simulink model "gm_DUALportRAMinterface_v3"  (R2024a)
settings: Solver=FixedStepDiscrete  StartTime=0.0  StopTime=20  RelTol=1e-3
undefined symbols (not defined in the file or in its folder): magnitude, Ts
libraries: hdlsllib x226, hdlmdlgenlib x102, embmathops x6, simulink x1, dsphdlxfrm2 x1
(part 1 of 6)
settings Model: Creator=Simon  LastModifiedBy=Simon
settings OptimizationCC: BlockReduction=off  ConditionallyExecuteInputs=off  DefaultParameterBehavior=Inlined  InheritOutputTypeSmallerThanSingle=on
settings DebuggingCC: AlgebraicLoopMsg=error  InheritedTsInSrcMsg=none  SingleTaskRateTransMsg=error  UnconnectedInputMsg=warning  UnconnectedOutputMsg=warning  UnconnectedLineMsg=warning
settings HardwareCC: ProdBitPerPointer=32  ProdBitPerSizeT=32  ProdBitPerPtrDiffT=32  ProdLargestAtomicFloat=None  ProdIntDivRoundTo=Undefined  ProdEndianess=Unspecified  ProdWordSize=32  ProdHWDeviceType=ASIC/FPGA->ASIC/FPGA  TargetBitPerPointer=64  TargetBitPerSizeT=64  TargetBitPerPtrDiffT=64  TargetLongLongMode=on  TargetIntDivRoundTo=Zero  TargetEndianess=LittleEndian  TargetWordSize=64  TargetHWDeviceType=Custom Processor->MATLAB Host Computer  ProdEqTarget=off

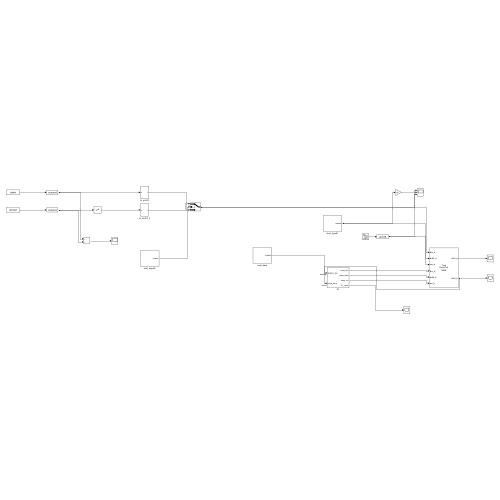
[thumbnail: Simulink's stored preview of the top-level diagram]
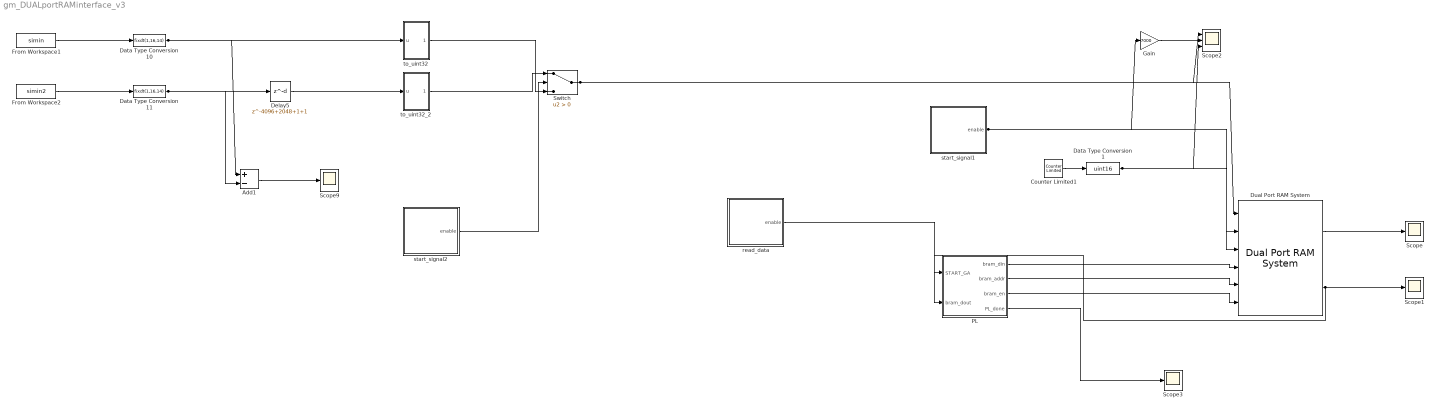
== system gm_DUALportRAMinterface_v3 ==
  Add1 : Sum  Inputs=+-
  Counter Limited1 : simulink/Sources/Counter Limited  uplimit=14000  tsamp=Ts
  Data Type Conversion1 : DataTypeConversion  OutDataTypeStr=uint16  SaturateOnIntegerOverflow=off  RndMeth=Floor
  Data Type Conversion10 : DataTypeConversion  OutDataTypeStr=fixdt(1,16,14)  SaturateOnIntegerOverflow=off  RndMeth=Floor
  Data Type Conversion11 : DataTypeConversion  OutDataTypeStr=fixdt(1,16,14)  SaturateOnIntegerOverflow=off  RndMeth=Floor
  Delay5 : Delay  DelayLength=4096+2048+1+1  InitialCondition=0  SampleTime=Ts
  Dual Port RAM System : hdlsllib/HDL RAMs/Dual Port RAM System  RAMType=True dual port  AsyncRead=off  WriteOutputValue=New data  RAMInitialValue=0  allowBusInputs=off  WritesHaveOutput=on  NumReads=0  NumWrites=1  SimulateUsing=Code generation
  From Workspace1 : FromWorkspace  VariableName=simin  SampleTime=Ts
  From Workspace2 : FromWorkspace  VariableName=simin2  SampleTime=Ts
  Gain : Gain  Gain=7000
  PL : Subsystem
  Scope{,1,3,9} (4 alike) : Scope
  Scope2 : Scope  NumInputPorts=3
  Switch : Switch  Criteria=u2 > Threshold  SaturateOnIntegerOverflow=off  InputSameDT=off  OutDataTypeStr=Inherit: Same as first input
  read_data : Subsystem
  start_signal1 : Subsystem
  start_signal2 : Subsystem
  to_uint32 : Subsystem
  to_uint32_2 : Subsystem
  wires:
  PL/4(PL_done) -> Scope3/1
  Data Type Conversion10/1 -> to_uint32/1(u), Add1/1
  Add1/1 -> Scope9/1
  Data Type Conversion11/1 -> Add1/2, Delay5/1
  Switch/1 -> Dual Port RAM System/1, Scope2/1
  Delay5/1 -> to_uint32_2/1(u)
  start_signal2/1(enable) -> Switch/2
  to_uint32_2/1(Out1) -> Switch/1
  to_uint32/1(Out1) -> Switch/3
  From Workspace2/1 -> Data Type Conversion11/1
  From Workspace1/1 -> Data Type Conversion10/1
  Dual Port RAM System/2 -> PL/2(bram_dout), Scope1/1
  read_data/1(enable) -> PL/1(START_GA)
  Gain/1 -> Scope2/2
  PL/3(bram_en) -> Dual Port RAM System/6
  PL/2(bram_addr) -> Dual Port RAM System/5
  PL/1(bram_din) -> Dual Port RAM System/4
  start_signal1/1(enable) -> Gain/1, Dual Port RAM System/3
  Data Type Conversion1/1 -> Dual Port RAM System/2, Scope2/3
  Counter Limited1/1 -> Data Type Conversion1/1
  Dual Port RAM System/1 -> Scope/1

== system gm_DUALportRAMinterface_v3/PL ==
  START_GA : Inport  OutDataTypeStr=boolean  PortDimensions=1  SampleTime=3.00000003e-08
  bram_dout : Inport  Port=2  OutDataTypeStr=uint32  PortDimensions=1  SampleTime=3.00000003e-08
  Bit Shift18 : hdlsllib/Logic and Bit Operations/Bit Shift  mode=Shift Right Logical  N=double(14)
  Chart : Subsystem
  Data Type Conversion2 : DataTypeConversion  OutDataTypeStr=uint32  SampleTime=3.00000003e-08  SaturateOnIntegerOverflow=off  RndMeth=Floor
  Data Type Conversion8 : DataTypeConversion  OutDataTypeStr=fixdt(0, 30, 14)  SampleTime=3.00000003e-08  SaturateOnIntegerOverflow=off  RndMeth=Floor
  Data Type Conversion9 : DataTypeConversion  OutDataTypeStr=fixdt(1, 16, 14)  SampleTime=3.00000003e-08  SaturateOnIntegerOverflow=off  RndMeth=Floor
  Delay : Delay  DelayLength=double(16)  InitialCondition=0  SampleTime=3.00000003e-08
  From{1..4,6,10..11} (7 alike) : hdlmdlgenlib/Buffer
  Goto{,1..5} (6 alike) : hdlmdlgenlib/Buffer
  Multiport Switch : MultiPortSwitch  DataPortOrder=Specify indices  Inputs=8  DataPortIndices={ double(0) double(1) double(2) double(3) double(4) double(5) double(6) double(7)}  DataPortForDefault=Additional data port  DiagnosticForDefault=None  OutDataTypeStr=uint32  SampleTime=3.00000003e-08  SaturateOnIntegerOverflow=off  InputSameDT=off
  index_counter : Subsystem
  integration_block1 : Subsystem
  t : Demux  Outputs=7
  to_uint32_1 : Subsystem
  to_uint32_2 : Subsystem
  to_uint32_3 : Subsystem
  to_uint32_4 : Subsystem
  to_uint32_5 : Subsystem
  to_uint32_6 : Subsystem
  bram_din : Outport  SampleTime=3.00000003e-08
  bram_addr : Outport  Port=2  SampleTime=3.00000003e-08
  bram_en : Outport  Port=3  SampleTime=3.00000003e-08
  PL_done : Outport  Port=4  SampleTime=3.00000003e-08
  wires:
  START_GA/1 -> integration_block1/3(start_ga), Chart/2(GPIO)
  bram_dout/1 -> Data Type Conversion8/1
  Bit Shift18/1 -> Data Type Conversion9/1
  Chart/3(write_enable) -> Goto4/1
  Data Type Conversion2/1 -> Multiport Switch/10, Multiport Switch/9, Multiport Switch/2
  Data Type Conversion8/1 -> Bit Shift18/1
  Data Type Conversion9/1 -> integration_block1/1(data_in), integration_block1/2(data_in1)
  Delay/1 -> Goto3/1
  From1/1 -> bram_addr/1
  From2/1 -> bram_en/1
  From3/1 -> PL_done/1
  From4/1 -> bram_din/1
  From6/1 -> Multiport Switch/1
  Multiport Switch/1 -> Goto/1
  index_counter/1(index_counter) -> Goto5/1, Chart/3(counter)
  integration_block1/1(ga_done) -> Delay/1, Chart/1(GA_done)
  integration_block1/2(elite_individual) -> t/1
  to_uint32_1/1(Out1) -> Multiport Switch/3
  to_uint32_2/1(Out1) -> Multiport Switch/4
  to_uint32_3/1(Out1) -> Multiport Switch/5
  to_uint32_4/1(Out1) -> Multiport Switch/6
  to_uint32_5/1(Out1) -> Multiport Switch/7
  to_uint32_6/1(Out1) -> Multiport Switch/8
  Goto5/1 -> From6/1, From1/1
  Goto4/1 -> From2/1
  Goto3/1 -> From3/1
  Goto/1 -> From4/1
  t/1 -> Data Type Conversion2/1
  t/2 -> to_uint32_1/1(u_port)
  t/3 -> to_uint32_2/1(u_port)
  t/4 -> to_uint32_3/1(u_port)
  t/5 -> to_uint32_4/1(u_port)
  t/6 -> to_uint32_5/1(u_port)
  t/7 -> to_uint32_6/1(u_port)
  From10/1 -> index_counter/2(In2)
  From11/1 -> index_counter/1(In1)
  Goto2/1 -> From10/1
  Goto1/1 -> From11/1
  Chart/1(counter_increment) -> Goto1/1
  Chart/2(counter_reset) -> Goto2/1

== system gm_DUALportRAMinterface_v3/read_data ==
  Data Type Conversion29 : DataTypeConversion  OutDataTypeStr=boolean  SaturateOnIntegerOverflow=off  RndMeth=Floor
  Delay2 : Delay  DelayLength=1  InitialCondition=0  SampleTime=Ts
  Gain : Gain
  Step1 : Step  Time=Ts*14000  SampleTime=Ts
  XOR1 : Logic  Operator=XOR  IconShape=distinctive  AllPortsSameDT=off  OutDataTypeStr=boolean
  enable : Outport
  wires:
  Data Type Conversion29/1 -> enable/1
  Gain/1 -> Data Type Conversion29/1
  Delay2/1 -> XOR1/2
  Step1/1 -> XOR1/1, Delay2/1
  XOR1/1 -> Gain/1

== system gm_DUALportRAMinterface_v3/start_signal1 ==
  Data Type Conversion29 : DataTypeConversion  OutDataTypeStr=boolean  SaturateOnIntegerOverflow=off  RndMeth=Floor
  Delay2 : Delay  DelayLength=(4096+2048+1+1)*2  InitialCondition=0  SampleTime=Ts
  Gain : Gain
  Step1 : Step  Time=Ts*0  SampleTime=Ts
  XOR1 : Logic  Operator=XOR  IconShape=distinctive  AllPortsSameDT=off  OutDataTypeStr=boolean
  enable : Outport
  wires:
  XOR1/1 -> Gain/1
  Step1/1 -> Delay2/1, XOR1/1
  Delay2/1 -> XOR1/2
  Gain/1 -> Data Type Conversion29/1
  Data Type Conversion29/1 -> enable/1

== system gm_DUALportRAMinterface_v3/start_signal2 ==
  Data Type Conversion29 : DataTypeConversion  OutDataTypeStr=boolean  SaturateOnIntegerOverflow=off  RndMeth=Floor
  Delay2 : Delay  DelayLength=(4096+2048+1+1)*2  InitialCondition=0  SampleTime=Ts
  Gain : Gain
  Step1 : Step  Time=Ts*(4096+2048+1+1)  SampleTime=Ts
  XOR1 : Logic  Operator=XOR  IconShape=distinctive  AllPortsSameDT=off  OutDataTypeStr=boolean
  enable : Outport
  wires:
  Data Type Conversion29/1 -> enable/1
  Gain/1 -> Data Type Conversion29/1
  Delay2/1 -> XOR1/2
  Step1/1 -> XOR1/1, Delay2/1
  XOR1/1 -> Gain/1

== system gm_DUALportRAMinterface_v3/to_uint32 ==
  u : Inport
  Bit Concat2 : hdlsllib/Logic and Bit Operations/Bit Concat  numInputs=16
  Bit Shift19 : hdlsllib/Logic and Bit Operations/Bit Shift  mode=Shift Left Logical  N=1
  Bit Shift20 : hdlsllib/Logic and Bit Operations/Bit Shift  mode=Shift Left Logical  N=10
  Bit Shift21 : hdlsllib/Logic and Bit Operations/Bit Shift  mode=Shift Right Logical  N=1
  Bit Shift22 : hdlsllib/Logic and Bit Operations/Bit Shift  mode=Shift Left Logical  N=11
  Bit Shift23 : hdlsllib/Logic and Bit Operations/Bit Shift  mode=Shift Left Logical  N=12
  Bit Shift24 : hdlsllib/Logic and Bit Operations/Bit Shift  mode=Shift Left Logical  N=13
  Bit Shift25 : hdlsllib/Logic and Bit Operations/Bit Shift  mode=Shift Left Logical  N=14
  Bit Shift26 : hdlsllib/Logic and Bit Operations/Bit Shift  mode=Shift Left Logical  N=2
  Bit Shift27 : hdlsllib/Logic and Bit Operations/Bit Shift  mode=Shift Left Logical  N=3
  Bit Shift28 : hdlsllib/Logic and Bit Operations/Bit Shift  mode=Shift Left Logical  N=4
  Bit Shift29 : hdlsllib/Logic and Bit Operations/Bit Shift  mode=Shift Left Logical  N=5
  Bit Shift30 : hdlsllib/Logic and Bit Operations/Bit Shift  mode=Shift Left Logical  N=6
  Bit Shift31 : hdlsllib/Logic and Bit Operations/Bit Shift  mode=Shift Left Logical  N=7
  Bit Shift32 : hdlsllib/Logic and Bit Operations/Bit Shift  mode=Shift Left Logical  N=8
  Bit Shift33 : hdlsllib/Logic and Bit Operations/Bit Shift  mode=Shift Left Logical  N=9
  Data Type Conversion{12..16,26,34..43} (16 alike) : DataTypeConversion  OutDataTypeStr=fixdt(0,1,0)  SaturateOnIntegerOverflow=off  RndMeth=Floor
  Data Type Conversion44 : DataTypeConversion  OutDataTypeStr=uint32  SaturateOnIntegerOverflow=off  RndMeth=Floor
  Out1 : Outport
  wires:
  Data Type Conversion14/1 -> Bit Concat2/10
  Bit Concat2/1 -> Data Type Conversion44/1
  Bit Shift26/1 -> Data Type Conversion35/1
  Bit Shift21/1 -> Data Type Conversion13/1
  Bit Shift28/1 -> Data Type Conversion26/1
  Data Type Conversion37/1 -> Bit Concat2/16
  Bit Shift29/1 -> Data Type Conversion16/1
  Bit Shift23/1 -> Data Type Conversion39/1
  Data Type Conversion41/1 -> Bit Concat2/12
  Bit Shift24/1 -> Data Type Conversion38/1
  Bit Shift33/1 -> Data Type Conversion42/1
  Data Type Conversion16/1 -> Bit Concat2/7
  Data Type Conversion43/1 -> Bit Concat2/9
  Data Type Conversion34/1 -> Bit Concat2/5
  Data Type Conversion39/1 -> Bit Concat2/14
  Bit Shift32/1 -> Data Type Conversion14/1
  Data Type Conversion12/1 -> Bit Concat2/2
  Bit Shift30/1 -> Data Type Conversion15/1
  Data Type Conversion15/1 -> Bit Concat2/8
  Bit Shift25/1 -> Data Type Conversion37/1
  Data Type Conversion38/1 -> Bit Concat2/15
  Bit Shift19/1 -> Data Type Conversion36/1
  Data Type Conversion42/1 -> Bit Concat2/11
  Data Type Conversion35/1 -> Bit Concat2/4
  Data Type Conversion44/1 -> Out1/1
  Data Type Conversion26/1 -> Bit Concat2/6
  Bit Shift31/1 -> Data Type Conversion43/1
  Data Type Conversion40/1 -> Bit Concat2/13
  Data Type Conversion13/1 -> Bit Concat2/1
  Bit Shift20/1 -> Data Type Conversion41/1
  u/1 -> Bit Shift25/1, Bit Shift24/1, Bit Shift23/1, Bit Shift22/1, Bit Shift20/1, Bit Shift33/1, Bit Shift32/1, Bit Shift31/1, Bit Shift30/1, Bit Shift29/1, Bit Shift28/1, Bit Shift27/1, Bit Shift26/1, Bit Shift19/1, Data Type Conversion12/1, Bit Shift21/1
  Data Type Conversion36/1 -> Bit Concat2/3
  Bit Shift27/1 -> Data Type Conversion34/1
  Bit Shift22/1 -> Data Type Conversion40/1

== system gm_DUALportRAMinterface_v3/to_uint32_2 ==
  u : Inport
  Bit Concat2 : hdlsllib/Logic and Bit Operations/Bit Concat  numInputs=16
  Bit Shift19 : hdlsllib/Logic and Bit Operations/Bit Shift  mode=Shift Left Logical  N=1
  Bit Shift20 : hdlsllib/Logic and Bit Operations/Bit Shift  mode=Shift Left Logical  N=10
  Bit Shift21 : hdlsllib/Logic and Bit Operations/Bit Shift  mode=Shift Right Logical  N=1
  Bit Shift22 : hdlsllib/Logic and Bit Operations/Bit Shift  mode=Shift Left Logical  N=11
  Bit Shift23 : hdlsllib/Logic and Bit Operations/Bit Shift  mode=Shift Left Logical  N=12
  Bit Shift24 : hdlsllib/Logic and Bit Operations/Bit Shift  mode=Shift Left Logical  N=13
  Bit Shift25 : hdlsllib/Logic and Bit Operations/Bit Shift  mode=Shift Left Logical  N=14
  Bit Shift26 : hdlsllib/Logic and Bit Operations/Bit Shift  mode=Shift Left Logical  N=2
  Bit Shift27 : hdlsllib/Logic and Bit Operations/Bit Shift  mode=Shift Left Logical  N=3
  Bit Shift28 : hdlsllib/Logic and Bit Operations/Bit Shift  mode=Shift Left Logical  N=4
  Bit Shift29 : hdlsllib/Logic and Bit Operations/Bit Shift  mode=Shift Left Logical  N=5
  Bit Shift30 : hdlsllib/Logic and Bit Operations/Bit Shift  mode=Shift Left Logical  N=6
  Bit Shift31 : hdlsllib/Logic and Bit Operations/Bit Shift  mode=Shift Left Logical  N=7
  Bit Shift32 : hdlsllib/Logic and Bit Operations/Bit Shift  mode=Shift Left Logical  N=8
  Bit Shift33 : hdlsllib/Logic and Bit Operations/Bit Shift  mode=Shift Left Logical  N=9
  Data Type Conversion{12..16,26,34..43} (16 alike) : DataTypeConversion  OutDataTypeStr=fixdt(0,1,0)  SaturateOnIntegerOverflow=off  RndMeth=Floor
  Data Type Conversion44 : DataTypeConversion  OutDataTypeStr=uint32  SaturateOnIntegerOverflow=off  RndMeth=Floor
  Out1 : Outport
  wires:
  Bit Shift22/1 -> Data Type Conversion40/1
  Bit Shift27/1 -> Data Type Conversion34/1
  Data Type Conversion36/1 -> Bit Concat2/3
  u/1 -> Bit Shift21/1, Data Type Conversion12/1, Bit Shift19/1, Bit Shift26/1, Bit Shift27/1, Bit Shift28/1, Bit Shift29/1, Bit Shift30/1, Bit Shift31/1, Bit Shift32/1, Bit Shift33/1, Bit Shift20/1, Bit Shift22/1, Bit Shift23/1, Bit Shift24/1, Bit Shift25/1
  Bit Shift20/1 -> Data Type Conversion41/1
  Data Type Conversion13/1 -> Bit Concat2/1
  Data Type Conversion40/1 -> Bit Concat2/13
  Bit Shift31/1 -> Data Type Conversion43/1
  Data Type Conversion26/1 -> Bit Concat2/6
  Data Type Conversion44/1 -> Out1/1
  Data Type Conversion35/1 -> Bit Concat2/4
  Data Type Conversion42/1 -> Bit Concat2/11
  Bit Shift19/1 -> Data Type Conversion36/1
  Data Type Conversion38/1 -> Bit Concat2/15
  Bit Shift25/1 -> Data Type Conversion37/1
  Data Type Conversion15/1 -> Bit Concat2/8
  Bit Shift30/1 -> Data Type Conversion15/1
  Data Type Conversion12/1 -> Bit Concat2/2
  Bit Shift32/1 -> Data Type Conversion14/1
  Data Type Conversion39/1 -> Bit Concat2/14
  Data Type Conversion34/1 -> Bit Concat2/5
  Data Type Conversion43/1 -> Bit Concat2/9
  Data Type Conversion16/1 -> Bit Concat2/7
  Bit Shift33/1 -> Data Type Conversion42/1
  Bit Shift24/1 -> Data Type Conversion38/1
  Data Type Conversion41/1 -> Bit Concat2/12
  Bit Shift23/1 -> Data Type Conversion39/1
  Bit Shift29/1 -> Data Type Conversion16/1
  Data Type Conversion37/1 -> Bit Concat2/16
  Bit Shift28/1 -> Data Type Conversion26/1
  Bit Shift21/1 -> Data Type Conversion13/1
  Bit Shift26/1 -> Data Type Conversion35/1
  Bit Concat2/1 -> Data Type Conversion44/1
  Data Type Conversion14/1 -> Bit Concat2/10

== system gm_DUALportRAMinterface_v3/PL/Chart ==
  GA_done : Inport  OutDataTypeStr=boolean  PortDimensions=1  SampleTime=3.00000003e-08
  GPIO : Inport  Port=2  OutDataTypeStr=boolean  PortDimensions=1  SampleTime=3.00000003e-08
  counter : Inport  Port=3  OutDataTypeStr=uint16  PortDimensions=1  SampleTime=3.00000003e-08
  Chart : Stateflow chart  TreatAsAtomicUnit=on
      settings: PortSchema="{\"entries\":[{\"content\":{\"sides\":[{\"content\":{\"connectorIds\":[\"In2\",\"In3\"]},\"type\":\"ConnectorPlacement.EquallySpacedRectSide\",\"uuid\":\"f3ce331f-c708-4668-a9cb-fb327ea74ab5\"},{\"content\":{\"connectorIds\":[\"Out1\",\"Out2\",\"Out3\"],\"side\":\"RIGHT\"},\"type\":\"ConnectorPlacement.EquallySpacedRectSide\",\"uuid\":\"3766927a-abff-497d-9544-2098881ba174\"},{\"content\":{\"side\":\"TOP\"},\"type\":\"ConnectorPlacement.EquallySpacedRectSide\",\"uuid\":\"ebfe3d64-ee7d-4953-a6ba-e7e40988decf\"},{\"content\":{\"connectorIds\":[\"In1\"],\"side\":\"BOTTOM\"},\"type\":\"ConnectorPlacement.EquallySpacedRectSide\",\"uuid\":\"f39ceaf8-4df7-4e40-9de5-da7597831fb4\"}]},\"type\":\"ConnectorPlacement.EquallySpacedConnector\",\"uuid\":\"89f60450-5933-42bb-b72b-5f8ec55483e0\"}],\"packageUris\":[\"http://schema.mathworks.com/mf0/Connector/R2020b\"],\"version\":\"1.0\"}"
  counter_increment : Outport  SampleTime=3.00000003e-08
  counter_reset : Outport  Port=2  SampleTime=3.00000003e-08
  write_enable : Outport  Port=3  SampleTime=3.00000003e-08
  wires:
  GA_done/1 -> Chart/1(GA_done)
  GPIO/1 -> Chart/2(GPIO)
  counter/1 -> Chart/3(counter)
  Chart/1(counter_increment) -> counter_increment/1
  Chart/2(counter_reset) -> counter_reset/1
  Chart/3(write_enable) -> write_enable/1

== system gm_DUALportRAMinterface_v3/PL/index_counter ==
  In1 : Inport  OutDataTypeStr=boolean  PortDimensions=1  SampleTime=3.00000003e-08
  In2 : Inport  Port=2  OutDataTypeStr=boolean  PortDimensions=1  SampleTime=3.00000003e-08
  Add : Sum  OutDataTypeStr=uint16
  Constant18 : Constant  OutDataTypeStr=fixdt(0,16,0)  SampleTime=Ts
  Constant19 : Constant  Value=0  OutDataTypeStr=fixdt(0,16,0)  SampleTime=Ts
  Constant20 : Constant  Value=0  OutDataTypeStr=uint16  SampleTime=Ts
  Delay : Delay  DelayLength=1  InitialCondition=0  SampleTime=Ts
  Switch : Switch  Criteria=u2 > Threshold  OutDataTypeStr=uint16  SaturateOnIntegerOverflow=off  InputSameDT=off
  Switch8 : Switch  Criteria=u2 > Threshold  OutDataTypeStr=uint16  SaturateOnIntegerOverflow=off  InputSameDT=off
  index_counter : Outport  SampleTime=3.00000003e-08
  wires:
  In1/1 -> Switch/2
  Constant18/1 -> Switch/1
  Constant19/1 -> Switch/3
  Delay/1 -> index_counter/1, Switch8/3
  Constant20/1 -> Switch8/1
  In2/1 -> Switch8/2
  Switch/1 -> Add/1
  Add/1 -> Delay/1
  Switch8/1 -> Add/2

== system gm_DUALportRAMinterface_v3/PL/integration_block1 ==
  data_in : Inport  OutDataTypeStr=fixdt(1, 16, 14)  PortDimensions=1  SampleTime=3.00000003e-08
  data_in1 : Inport  Port=2  OutDataTypeStr=fixdt(1, 16, 14)  PortDimensions=1  SampleTime=3.00000003e-08
  start_ga : Inport  Port=3  OutDataTypeStr=boolean  PortDimensions=1  SampleTime=3.00000003e-08
  D2 : Subsystem
  Delay : Delay  DelayLength=double(6145)  InitialCondition=0  SampleTime=3.00000003e-08
  Delay3 : Delay  DelayLength=double(1)  InitialCondition=0  SampleTime=3.00000003e-08
  FFT : dsphdlxfrm2/FFT  Architecture=Burst Radix 2  FFTLengthSource=Property  FFTLength=4096  FFTLengthMax=1024  ComplexMultiplication=Use 4 multipliers and 2 adders  BitReversedOutput=off  BitReversedInput=off  Normalize=off  SimulateUsing=Code generation  RoundingMethod=Floor  ResetInputPort=on  StartOutputPort=off  EndOutputPort=off
  FFT_term2 : Terminator
  FIFO_system1 : Subsystem
  FIFO_system3 : Subsystem
  FIFO_system3_term1 : Terminator
  FIFO_system3_term2 : Terminator
  GA_main : Subsystem
  Subsystem : Subsystem
  Sum : Sum  Inputs=+-  OutDataTypeStr=fixdt(1, 16, 14)  AccumDataTypeStr=fixdt(1, 16, 14)  SampleTime=3.00000003e-08
  accumulator_scorer : Subsystem
  ga_done : Outport  SampleTime=3.00000003e-08
  elite_individual : Outport  Port=2  SampleTime=3.00000003e-08
  wires:
  start_ga/1 -> Subsystem/1(enable), GA_main/1(start_ga)
  FFT/3 -> FFT_term2/1
  GA_main/1(elite_individual) -> elite_individual/1
  GA_main/2(ga_done) -> ga_done/1
  FIFO_system3/2(data_valid) -> FIFO_system3_term1/1
  FIFO_system3/3(reset_fft) -> FIFO_system3_term2/1
  GA_main/4(FIFO_out_en) -> FIFO_system3/2(enable_output), FIFO_system1/2(enable_output), D2/2(push_individual)
  FIFO_system1/3(reset_fft) -> Delay/1, FFT/3
  accumulator_scorer/1(individual_score) -> GA_main/2(score_result)
  accumulator_scorer/2(individual_score_valid) -> Delay3/1
  GA_main/3(individual_to_d2) -> D2/4(Individual_input)
  GA_main/5(load_fifo) -> FIFO_system1/3(load_fifo)
  Subsystem/1(random_gene_out) -> GA_main/3(random_gene)
  Subsystem/2(random_method_out) -> GA_main/4(random_method)
  Subsystem/3(b2_random_out) -> GA_main/5(b2rnd)
  Subsystem/4(b3_random_out) -> GA_main/6(b3rnd)
  Subsystem/5(b4_random_out) -> GA_main/7(b4rnd)
  Subsystem/6(a2_random_out) -> GA_main/8(a2rnd)
  Subsystem/7(a3_random_out) -> GA_main/9(a3rnd)
  Subsystem/8(a4_random_out) -> GA_main/10(a4rnd)
  Subsystem/9(random_sample_out) -> GA_main/11(tb_random_sample)
  Delay3/1 -> GA_main/13(score_done)
  D2/1(response) -> Sum/2
  FIFO_system3/1(data_out) -> D2/1(GAerror)
  FIFO_system3/4(FIFO_full) -> GA_main/12(FIFO_full)
  data_in1/1 -> FIFO_system3/1(data_in)
  FIFO_system1/1(data_out) -> Sum/1
  FIFO_system1/2(data_valid) -> FFT/2
  FIFO_system1/4(FIFO_full) -> FIFO_system3/3(load_fifo)
  data_in/1 -> FIFO_system1/1(data_in)
  Delay/1 -> D2/3(reset_D2)
  FFT/1 -> accumulator_scorer/1(data_in)
  FFT/2 -> accumulator_scorer/2(valid_fft)
  Sum/1 -> FFT/1

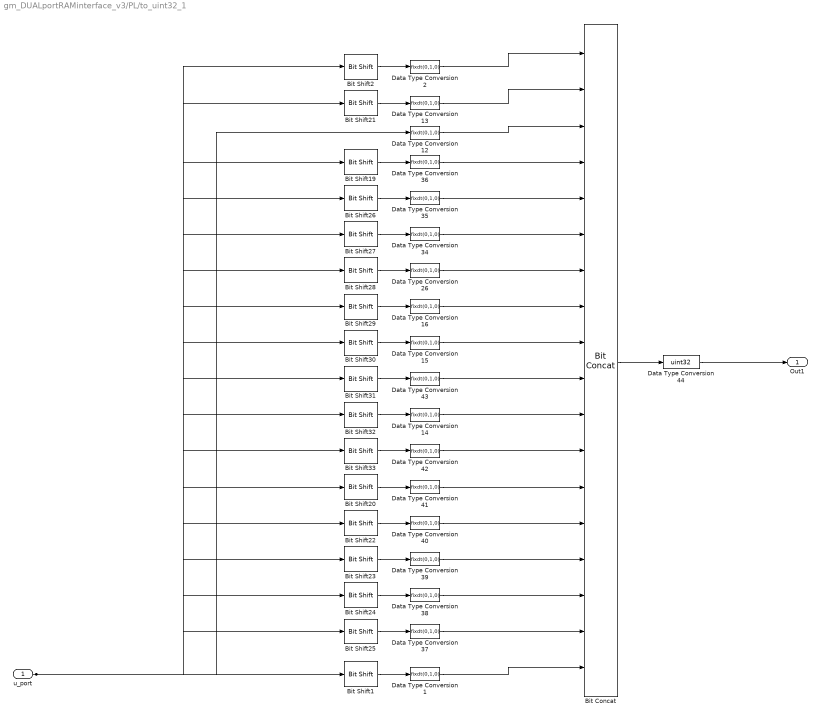
== system gm_DUALportRAMinterface_v3/PL/to_uint32_1 ==
  u_port : Inport  OutDataTypeStr=fixdt(1, 33, 15)  PortDimensions=1  SampleTime=3.00000003e-08
  Bit Concat : hdlsllib/Logic and Bit Operations/Bit Concat  numInputs=18
  Bit Shift1 : hdlsllib/Logic and Bit Operations/Bit Shift  mode=Shift Left Logical  N=15
  Bit Shift19 : hdlsllib/Logic and Bit Operations/Bit Shift  mode=Shift Left Logical  N=1
  Bit Shift2 : hdlsllib/Logic and Bit Operations/Bit Shift  mode=Shift Right Logical  N=16
  Bit Shift20 : hdlsllib/Logic and Bit Operations/Bit Shift  mode=Shift Left Logical  N=10
  Bit Shift21 : hdlsllib/Logic and Bit Operations/Bit Shift  mode=Shift Right Logical  N=1
  Bit Shift22 : hdlsllib/Logic and Bit Operations/Bit Shift  mode=Shift Left Logical  N=11
  Bit Shift23 : hdlsllib/Logic and Bit Operations/Bit Shift  mode=Shift Left Logical  N=12
  Bit Shift24 : hdlsllib/Logic and Bit Operations/Bit Shift  mode=Shift Left Logical  N=13
  Bit Shift25 : hdlsllib/Logic and Bit Operations/Bit Shift  mode=Shift Left Logical  N=14
  Bit Shift26 : hdlsllib/Logic and Bit Operations/Bit Shift  mode=Shift Left Logical  N=2
  Bit Shift27 : hdlsllib/Logic and Bit Operations/Bit Shift  mode=Shift Left Logical  N=3
  Bit Shift28 : hdlsllib/Logic and Bit Operations/Bit Shift  mode=Shift Left Logical  N=4
  Bit Shift29 : hdlsllib/Logic and Bit Operations/Bit Shift  mode=Shift Left Logical  N=5
  Bit Shift30 : hdlsllib/Logic and Bit Operations/Bit Shift  mode=Shift Left Logical  N=6
  Bit Shift31 : hdlsllib/Logic and Bit Operations/Bit Shift  mode=Shift Left Logical  N=7
  Bit Shift32 : hdlsllib/Logic and Bit Operations/Bit Shift  mode=Shift Left Logical  N=8
  Bit Shift33 : hdlsllib/Logic and Bit Operations/Bit Shift  mode=Shift Left Logical  N=9
  Data Type Conversion{1..2,12..16,26,34..43} (18 alike) : DataTypeConversion  OutDataTypeStr=fixdt(0,1,0)  SaturateOnIntegerOverflow=off  RndMeth=Floor
  Data Type Conversion44 : DataTypeConversion  OutDataTypeStr=uint32  SaturateOnIntegerOverflow=off  RndMeth=Floor
  Out1 : Outport  SampleTime=3.00000003e-08
  wires:
  u_port/1 -> Data Type Conversion12/1, Bit Shift33/1, Bit Shift32/1, Bit Shift31/1, Bit Shift30/1, Bit Shift29/1, Bit Shift28/1, Bit Shift27/1, Bit Shift26/1, Bit Shift25/1, Bit Shift24/1, Bit Shift23/1, Bit Shift22/1, Bit Shift21/1, Bit Shift20/1, Bit Shift2/1, Bit Shift19/1, Bit Shift1/1
  Bit Concat/1 -> Data Type Conversion44/1
  Bit Shift1/1 -> Data Type Conversion1/1
  Bit Shift19/1 -> Data Type Conversion36/1
  Bit Shift2/1 -> Data Type Conversion2/1
  Bit Shift20/1 -> Data Type Conversion41/1
  Bit Shift21/1 -> Data Type Conversion13/1
  Bit Shift22/1 -> Data Type Conversion40/1
  Bit Shift23/1 -> Data Type Conversion39/1
  Bit Shift24/1 -> Data Type Conversion38/1
  Bit Shift25/1 -> Data Type Conversion37/1
  Bit Shift26/1 -> Data Type Conversion35/1
  Bit Shift27/1 -> Data Type Conversion34/1
  Bit Shift28/1 -> Data Type Conversion26/1
  Bit Shift29/1 -> Data Type Conversion16/1
  Bit Shift30/1 -> Data Type Conversion15/1
  Bit Shift31/1 -> Data Type Conversion43/1
  Bit Shift32/1 -> Data Type Conversion14/1
  Bit Shift33/1 -> Data Type Conversion42/1
  Data Type Conversion1/1 -> Bit Concat/18
  Data Type Conversion12/1 -> Bit Concat/3
  Data Type Conversion13/1 -> Bit Concat/2
  Data Type Conversion14/1 -> Bit Concat/11
  Data Type Conversion15/1 -> Bit Concat/9
  Data Type Conversion16/1 -> Bit Concat/8
  Data Type Conversion2/1 -> Bit Concat/1
  Data Type Conversion26/1 -> Bit Concat/7
  Data Type Conversion34/1 -> Bit Concat/6
  Data Type Conversion35/1 -> Bit Concat/5
  Data Type Conversion36/1 -> Bit Concat/4
  Data Type Conversion37/1 -> Bit Concat/17
  Data Type Conversion38/1 -> Bit Concat/16
  Data Type Conversion39/1 -> Bit Concat/15
  Data Type Conversion40/1 -> Bit Concat/14
  Data Type Conversion41/1 -> Bit Concat/13
  Data Type Conversion42/1 -> Bit Concat/12
  Data Type Conversion43/1 -> Bit Concat/10
  Data Type Conversion44/1 -> Out1/1

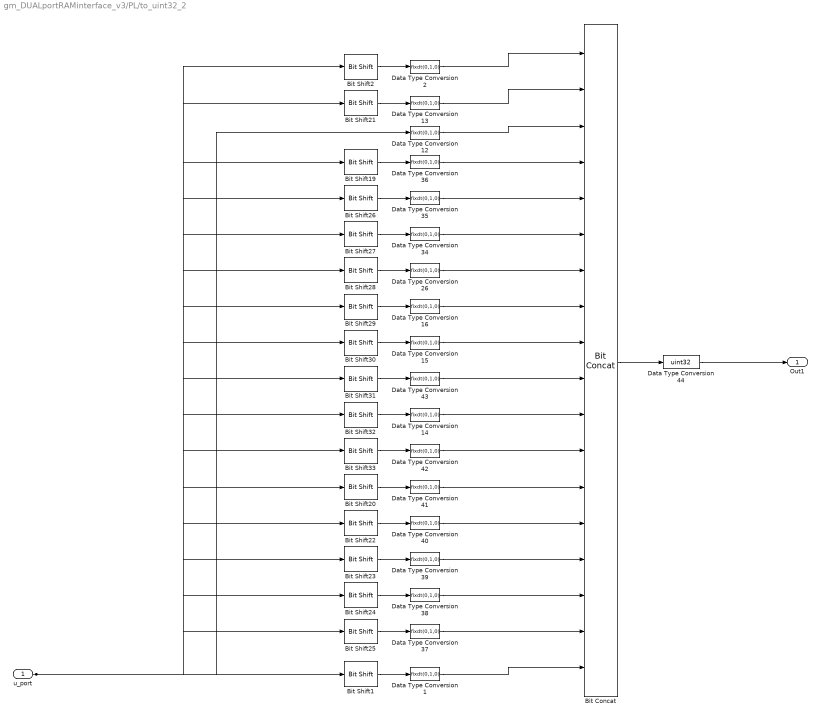
== system gm_DUALportRAMinterface_v3/PL/to_uint32_2 ==
  u_port : Inport  OutDataTypeStr=fixdt(1, 33, 15)  PortDimensions=1  SampleTime=3.00000003e-08
  Bit Concat : hdlsllib/Logic and Bit Operations/Bit Concat  numInputs=18
  Bit Shift1 : hdlsllib/Logic and Bit Operations/Bit Shift  mode=Shift Left Logical  N=15
  Bit Shift19 : hdlsllib/Logic and Bit Operations/Bit Shift  mode=Shift Left Logical  N=1
  Bit Shift2 : hdlsllib/Logic and Bit Operations/Bit Shift  mode=Shift Right Logical  N=16
  Bit Shift20 : hdlsllib/Logic and Bit Operations/Bit Shift  mode=Shift Left Logical  N=10
  Bit Shift21 : hdlsllib/Logic and Bit Operations/Bit Shift  mode=Shift Right Logical  N=1
  Bit Shift22 : hdlsllib/Logic and Bit Operations/Bit Shift  mode=Shift Left Logical  N=11
  Bit Shift23 : hdlsllib/Logic and Bit Operations/Bit Shift  mode=Shift Left Logical  N=12
  Bit Shift24 : hdlsllib/Logic and Bit Operations/Bit Shift  mode=Shift Left Logical  N=13
  Bit Shift25 : hdlsllib/Logic and Bit Operations/Bit Shift  mode=Shift Left Logical  N=14
  Bit Shift26 : hdlsllib/Logic and Bit Operations/Bit Shift  mode=Shift Left Logical  N=2
  Bit Shift27 : hdlsllib/Logic and Bit Operations/Bit Shift  mode=Shift Left Logical  N=3
  Bit Shift28 : hdlsllib/Logic and Bit Operations/Bit Shift  mode=Shift Left Logical  N=4
  Bit Shift29 : hdlsllib/Logic and Bit Operations/Bit Shift  mode=Shift Left Logical  N=5
  Bit Shift30 : hdlsllib/Logic and Bit Operations/Bit Shift  mode=Shift Left Logical  N=6
  Bit Shift31 : hdlsllib/Logic and Bit Operations/Bit Shift  mode=Shift Left Logical  N=7
  Bit Shift32 : hdlsllib/Logic and Bit Operations/Bit Shift  mode=Shift Left Logical  N=8
  Bit Shift33 : hdlsllib/Logic and Bit Operations/Bit Shift  mode=Shift Left Logical  N=9
  Data Type Conversion{1..2,12..16,26,34..43} (18 alike) : DataTypeConversion  OutDataTypeStr=fixdt(0,1,0)  SaturateOnIntegerOverflow=off  RndMeth=Floor
  Data Type Conversion44 : DataTypeConversion  OutDataTypeStr=uint32  SaturateOnIntegerOverflow=off  RndMeth=Floor
  Out1 : Outport  SampleTime=3.00000003e-08
  wires:
  u_port/1 -> Data Type Conversion12/1, Bit Shift33/1, Bit Shift32/1, Bit Shift31/1, Bit Shift30/1, Bit Shift29/1, Bit Shift28/1, Bit Shift27/1, Bit Shift26/1, Bit Shift25/1, Bit Shift24/1, Bit Shift23/1, Bit Shift22/1, Bit Shift21/1, Bit Shift20/1, Bit Shift2/1, Bit Shift19/1, Bit Shift1/1
  Bit Concat/1 -> Data Type Conversion44/1
  Bit Shift1/1 -> Data Type Conversion1/1
  Bit Shift19/1 -> Data Type Conversion36/1
  Bit Shift2/1 -> Data Type Conversion2/1
  Bit Shift20/1 -> Data Type Conversion41/1
  Bit Shift21/1 -> Data Type Conversion13/1
  Bit Shift22/1 -> Data Type Conversion40/1
  Bit Shift23/1 -> Data Type Conversion39/1
  Bit Shift24/1 -> Data Type Conversion38/1
  Bit Shift25/1 -> Data Type Conversion37/1
  Bit Shift26/1 -> Data Type Conversion35/1
  Bit Shift27/1 -> Data Type Conversion34/1
  Bit Shift28/1 -> Data Type Conversion26/1
  Bit Shift29/1 -> Data Type Conversion16/1
  Bit Shift30/1 -> Data Type Conversion15/1
  Bit Shift31/1 -> Data Type Conversion43/1
  Bit Shift32/1 -> Data Type Conversion14/1
  Bit Shift33/1 -> Data Type Conversion42/1
  Data Type Conversion1/1 -> Bit Concat/18
  Data Type Conversion12/1 -> Bit Concat/3
  Data Type Conversion13/1 -> Bit Concat/2
  Data Type Conversion14/1 -> Bit Concat/11
  Data Type Conversion15/1 -> Bit Concat/9
  Data Type Conversion16/1 -> Bit Concat/8
  Data Type Conversion2/1 -> Bit Concat/1
  Data Type Conversion26/1 -> Bit Concat/7
  Data Type Conversion34/1 -> Bit Concat/6
  Data Type Conversion35/1 -> Bit Concat/5
  Data Type Conversion36/1 -> Bit Concat/4
  Data Type Conversion37/1 -> Bit Concat/17
  Data Type Conversion38/1 -> Bit Concat/16
  Data Type Conversion39/1 -> Bit Concat/15
  Data Type Conversion40/1 -> Bit Concat/14
  Data Type Conversion41/1 -> Bit Concat/13
  Data Type Conversion42/1 -> Bit Concat/12
  Data Type Conversion43/1 -> Bit Concat/10
  Data Type Conversion44/1 -> Out1/1

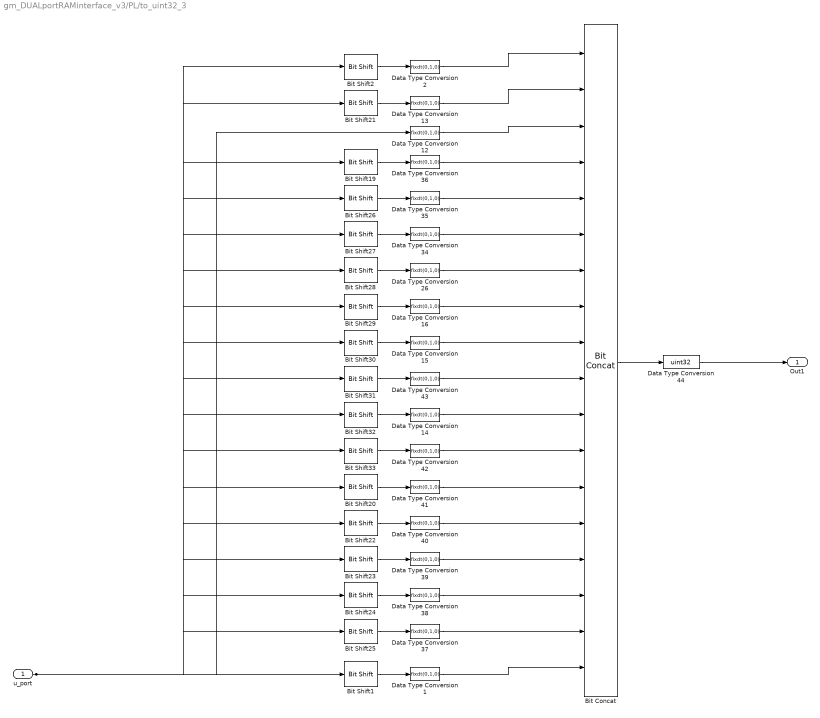
== system gm_DUALportRAMinterface_v3/PL/to_uint32_3 ==
  u_port : Inport  OutDataTypeStr=fixdt(1, 33, 15)  PortDimensions=1  SampleTime=3.00000003e-08
  Bit Concat : hdlsllib/Logic and Bit Operations/Bit Concat  numInputs=18
  Bit Shift1 : hdlsllib/Logic and Bit Operations/Bit Shift  mode=Shift Left Logical  N=15
  Bit Shift19 : hdlsllib/Logic and Bit Operations/Bit Shift  mode=Shift Left Logical  N=1
  Bit Shift2 : hdlsllib/Logic and Bit Operations/Bit Shift  mode=Shift Right Logical  N=16
  Bit Shift20 : hdlsllib/Logic and Bit Operations/Bit Shift  mode=Shift Left Logical  N=10
  Bit Shift21 : hdlsllib/Logic and Bit Operations/Bit Shift  mode=Shift Right Logical  N=1
  Bit Shift22 : hdlsllib/Logic and Bit Operations/Bit Shift  mode=Shift Left Logical  N=11
  Bit Shift23 : hdlsllib/Logic and Bit Operations/Bit Shift  mode=Shift Left Logical  N=12
  Bit Shift24 : hdlsllib/Logic and Bit Operations/Bit Shift  mode=Shift Left Logical  N=13
  Bit Shift25 : hdlsllib/Logic and Bit Operations/Bit Shift  mode=Shift Left Logical  N=14
  Bit Shift26 : hdlsllib/Logic and Bit Operations/Bit Shift  mode=Shift Left Logical  N=2
  Bit Shift27 : hdlsllib/Logic and Bit Operations/Bit Shift  mode=Shift Left Logical  N=3
  Bit Shift28 : hdlsllib/Logic and Bit Operations/Bit Shift  mode=Shift Left Logical  N=4
  Bit Shift29 : hdlsllib/Logic and Bit Operations/Bit Shift  mode=Shift Left Logical  N=5
  Bit Shift30 : hdlsllib/Logic and Bit Operations/Bit Shift  mode=Shift Left Logical  N=6
  Bit Shift31 : hdlsllib/Logic and Bit Operations/Bit Shift  mode=Shift Left Logical  N=7
  Bit Shift32 : hdlsllib/Logic and Bit Operations/Bit Shift  mode=Shift Left Logical  N=8
  Bit Shift33 : hdlsllib/Logic and Bit Operations/Bit Shift  mode=Shift Left Logical  N=9
  Data Type Conversion{1..2,12..16,26,34..43} (18 alike) : DataTypeConversion  OutDataTypeStr=fixdt(0,1,0)  SaturateOnIntegerOverflow=off  RndMeth=Floor
  Data Type Conversion44 : DataTypeConversion  OutDataTypeStr=uint32  SaturateOnIntegerOverflow=off  RndMeth=Floor
  Out1 : Outport  SampleTime=3.00000003e-08
  wires:
  u_port/1 -> Data Type Conversion12/1, Bit Shift33/1, Bit Shift32/1, Bit Shift31/1, Bit Shift30/1, Bit Shift29/1, Bit Shift28/1, Bit Shift27/1, Bit Shift26/1, Bit Shift25/1, Bit Shift24/1, Bit Shift23/1, Bit Shift22/1, Bit Shift21/1, Bit Shift20/1, Bit Shift2/1, Bit Shift19/1, Bit Shift1/1
  Bit Concat/1 -> Data Type Conversion44/1
  Bit Shift1/1 -> Data Type Conversion1/1
  Bit Shift19/1 -> Data Type Conversion36/1
  Bit Shift2/1 -> Data Type Conversion2/1
  Bit Shift20/1 -> Data Type Conversion41/1
  Bit Shift21/1 -> Data Type Conversion13/1
  Bit Shift22/1 -> Data Type Conversion40/1
  Bit Shift23/1 -> Data Type Conversion39/1
  Bit Shift24/1 -> Data Type Conversion38/1
  Bit Shift25/1 -> Data Type Conversion37/1
  Bit Shift26/1 -> Data Type Conversion35/1
  Bit Shift27/1 -> Data Type Conversion34/1
  Bit Shift28/1 -> Data Type Conversion26/1
  Bit Shift29/1 -> Data Type Conversion16/1
  Bit Shift30/1 -> Data Type Conversion15/1
  Bit Shift31/1 -> Data Type Conversion43/1
  Bit Shift32/1 -> Data Type Conversion14/1
  Bit Shift33/1 -> Data Type Conversion42/1
  Data Type Conversion1/1 -> Bit Concat/18
  Data Type Conversion12/1 -> Bit Concat/3
  Data Type Conversion13/1 -> Bit Concat/2
  Data Type Conversion14/1 -> Bit Concat/11
  Data Type Conversion15/1 -> Bit Concat/9
  Data Type Conversion16/1 -> Bit Concat/8
  Data Type Conversion2/1 -> Bit Concat/1
  Data Type Conversion26/1 -> Bit Concat/7
  Data Type Conversion34/1 -> Bit Concat/6
  Data Type Conversion35/1 -> Bit Concat/5
  Data Type Conversion36/1 -> Bit Concat/4
  Data Type Conversion37/1 -> Bit Concat/17
  Data Type Conversion38/1 -> Bit Concat/16
  Data Type Conversion39/1 -> Bit Concat/15
  Data Type Conversion40/1 -> Bit Concat/14
  Data Type Conversion41/1 -> Bit Concat/13
  Data Type Conversion42/1 -> Bit Concat/12
  Data Type Conversion43/1 -> Bit Concat/10
  Data Type Conversion44/1 -> Out1/1

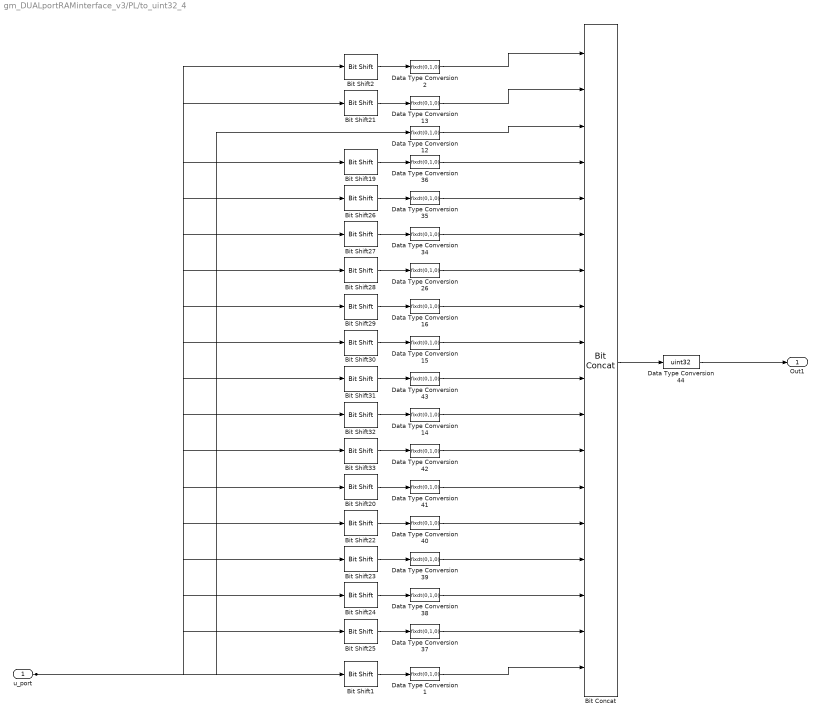
== system gm_DUALportRAMinterface_v3/PL/to_uint32_4 ==
  u_port : Inport  OutDataTypeStr=fixdt(1, 33, 15)  PortDimensions=1  SampleTime=3.00000003e-08
  Bit Concat : hdlsllib/Logic and Bit Operations/Bit Concat  numInputs=18
  Bit Shift1 : hdlsllib/Logic and Bit Operations/Bit Shift  mode=Shift Left Logical  N=15
  Bit Shift19 : hdlsllib/Logic and Bit Operations/Bit Shift  mode=Shift Left Logical  N=1
  Bit Shift2 : hdlsllib/Logic and Bit Operations/Bit Shift  mode=Shift Right Logical  N=16
  Bit Shift20 : hdlsllib/Logic and Bit Operations/Bit Shift  mode=Shift Left Logical  N=10
  Bit Shift21 : hdlsllib/Logic and Bit Operations/Bit Shift  mode=Shift Right Logical  N=1
  Bit Shift22 : hdlsllib/Logic and Bit Operations/Bit Shift  mode=Shift Left Logical  N=11
  Bit Shift23 : hdlsllib/Logic and Bit Operations/Bit Shift  mode=Shift Left Logical  N=12
  Bit Shift24 : hdlsllib/Logic and Bit Operations/Bit Shift  mode=Shift Left Logical  N=13
  Bit Shift25 : hdlsllib/Logic and Bit Operations/Bit Shift  mode=Shift Left Logical  N=14
  Bit Shift26 : hdlsllib/Logic and Bit Operations/Bit Shift  mode=Shift Left Logical  N=2
  Bit Shift27 : hdlsllib/Logic and Bit Operations/Bit Shift  mode=Shift Left Logical  N=3
  Bit Shift28 : hdlsllib/Logic and Bit Operations/Bit Shift  mode=Shift Left Logical  N=4
  Bit Shift29 : hdlsllib/Logic and Bit Operations/Bit Shift  mode=Shift Left Logical  N=5
  Bit Shift30 : hdlsllib/Logic and Bit Operations/Bit Shift  mode=Shift Left Logical  N=6
  Bit Shift31 : hdlsllib/Logic and Bit Operations/Bit Shift  mode=Shift Left Logical  N=7
  Bit Shift32 : hdlsllib/Logic and Bit Operations/Bit Shift  mode=Shift Left Logical  N=8
  Bit Shift33 : hdlsllib/Logic and Bit Operations/Bit Shift  mode=Shift Left Logical  N=9
  Data Type Conversion{1..2,12..16,26,34..43} (18 alike) : DataTypeConversion  OutDataTypeStr=fixdt(0,1,0)  SaturateOnIntegerOverflow=off  RndMeth=Floor
  Data Type Conversion44 : DataTypeConversion  OutDataTypeStr=uint32  SaturateOnIntegerOverflow=off  RndMeth=Floor
  Out1 : Outport  SampleTime=3.00000003e-08
  wires:
  u_port/1 -> Data Type Conversion12/1, Bit Shift33/1, Bit Shift32/1, Bit Shift31/1, Bit Shift30/1, Bit Shift29/1, Bit Shift28/1, Bit Shift27/1, Bit Shift26/1, Bit Shift25/1, Bit Shift24/1, Bit Shift23/1, Bit Shift22/1, Bit Shift21/1, Bit Shift20/1, Bit Shift2/1, Bit Shift19/1, Bit Shift1/1
  Bit Concat/1 -> Data Type Conversion44/1
  Bit Shift1/1 -> Data Type Conversion1/1
  Bit Shift19/1 -> Data Type Conversion36/1
  Bit Shift2/1 -> Data Type Conversion2/1
  Bit Shift20/1 -> Data Type Conversion41/1
  Bit Shift21/1 -> Data Type Conversion13/1
  Bit Shift22/1 -> Data Type Conversion40/1
  Bit Shift23/1 -> Data Type Conversion39/1
  Bit Shift24/1 -> Data Type Conversion38/1
  Bit Shift25/1 -> Data Type Conversion37/1
  Bit Shift26/1 -> Data Type Conversion35/1
  Bit Shift27/1 -> Data Type Conversion34/1
  Bit Shift28/1 -> Data Type Conversion26/1
  Bit Shift29/1 -> Data Type Conversion16/1
  Bit Shift30/1 -> Data Type Conversion15/1
  Bit Shift31/1 -> Data Type Conversion43/1
  Bit Shift32/1 -> Data Type Conversion14/1
  Bit Shift33/1 -> Data Type Conversion42/1
  Data Type Conversion1/1 -> Bit Concat/18
  Data Type Conversion12/1 -> Bit Concat/3
  Data Type Conversion13/1 -> Bit Concat/2
  Data Type Conversion14/1 -> Bit Concat/11
  Data Type Conversion15/1 -> Bit Concat/9
  Data Type Conversion16/1 -> Bit Concat/8
  Data Type Conversion2/1 -> Bit Concat/1
  Data Type Conversion26/1 -> Bit Concat/7
  Data Type Conversion34/1 -> Bit Concat/6
  Data Type Conversion35/1 -> Bit Concat/5
  Data Type Conversion36/1 -> Bit Concat/4
  Data Type Conversion37/1 -> Bit Concat/17
  Data Type Conversion38/1 -> Bit Concat/16
  Data Type Conversion39/1 -> Bit Concat/15
  Data Type Conversion40/1 -> Bit Concat/14
  Data Type Conversion41/1 -> Bit Concat/13
  Data Type Conversion42/1 -> Bit Concat/12
  Data Type Conversion43/1 -> Bit Concat/10
  Data Type Conversion44/1 -> Out1/1

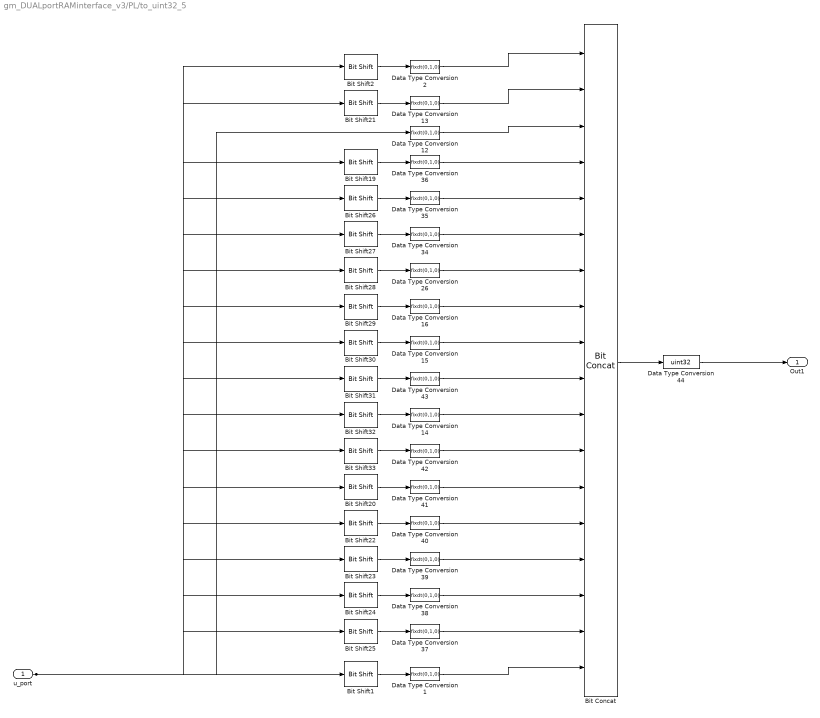
== system gm_DUALportRAMinterface_v3/PL/to_uint32_5 ==
  u_port : Inport  OutDataTypeStr=fixdt(1, 33, 15)  PortDimensions=1  SampleTime=3.00000003e-08
  Bit Concat : hdlsllib/Logic and Bit Operations/Bit Concat  numInputs=18
  Bit Shift1 : hdlsllib/Logic and Bit Operations/Bit Shift  mode=Shift Left Logical  N=15
  Bit Shift19 : hdlsllib/Logic and Bit Operations/Bit Shift  mode=Shift Left Logical  N=1
  Bit Shift2 : hdlsllib/Logic and Bit Operations/Bit Shift  mode=Shift Right Logical  N=16
  Bit Shift20 : hdlsllib/Logic and Bit Operations/Bit Shift  mode=Shift Left Logical  N=10
  Bit Shift21 : hdlsllib/Logic and Bit Operations/Bit Shift  mode=Shift Right Logical  N=1
  Bit Shift22 : hdlsllib/Logic and Bit Operations/Bit Shift  mode=Shift Left Logical  N=11
  Bit Shift23 : hdlsllib/Logic and Bit Operations/Bit Shift  mode=Shift Left Logical  N=12
  Bit Shift24 : hdlsllib/Logic and Bit Operations/Bit Shift  mode=Shift Left Logical  N=13
  Bit Shift25 : hdlsllib/Logic and Bit Operations/Bit Shift  mode=Shift Left Logical  N=14
  Bit Shift26 : hdlsllib/Logic and Bit Operations/Bit Shift  mode=Shift Left Logical  N=2
  Bit Shift27 : hdlsllib/Logic and Bit Operations/Bit Shift  mode=Shift Left Logical  N=3
  Bit Shift28 : hdlsllib/Logic and Bit Operations/Bit Shift  mode=Shift Left Logical  N=4
  Bit Shift29 : hdlsllib/Logic and Bit Operations/Bit Shift  mode=Shift Left Logical  N=5
  Bit Shift30 : hdlsllib/Logic and Bit Operations/Bit Shift  mode=Shift Left Logical  N=6
  Bit Shift31 : hdlsllib/Logic and Bit Operations/Bit Shift  mode=Shift Left Logical  N=7
  Bit Shift32 : hdlsllib/Logic and Bit Operations/Bit Shift  mode=Shift Left Logical  N=8
  Bit Shift33 : hdlsllib/Logic and Bit Operations/Bit Shift  mode=Shift Left Logical  N=9
  Data Type Conversion{1..2,12..16,26,34..43} (18 alike) : DataTypeConversion  OutDataTypeStr=fixdt(0,1,0)  SaturateOnIntegerOverflow=off  RndMeth=Floor
  Data Type Conversion44 : DataTypeConversion  OutDataTypeStr=uint32  SaturateOnIntegerOverflow=off  RndMeth=Floor
  Out1 : Outport  SampleTime=3.00000003e-08
  wires:
  u_port/1 -> Data Type Conversion12/1, Bit Shift33/1, Bit Shift32/1, Bit Shift31/1, Bit Shift30/1, Bit Shift29/1, Bit Shift28/1, Bit Shift27/1, Bit Shift26/1, Bit Shift25/1, Bit Shift24/1, Bit Shift23/1, Bit Shift22/1, Bit Shift21/1, Bit Shift20/1, Bit Shift2/1, Bit Shift19/1, Bit Shift1/1
  Bit Concat/1 -> Data Type Conversion44/1
  Bit Shift1/1 -> Data Type Conversion1/1
  Bit Shift19/1 -> Data Type Conversion36/1
  Bit Shift2/1 -> Data Type Conversion2/1
  Bit Shift20/1 -> Data Type Conversion41/1
  Bit Shift21/1 -> Data Type Conversion13/1
  Bit Shift22/1 -> Data Type Conversion40/1
  Bit Shift23/1 -> Data Type Conversion39/1
  Bit Shift24/1 -> Data Type Conversion38/1
  Bit Shift25/1 -> Data Type Conversion37/1
  Bit Shift26/1 -> Data Type Conversion35/1
  Bit Shift27/1 -> Data Type Conversion34/1
  Bit Shift28/1 -> Data Type Conversion26/1
  Bit Shift29/1 -> Data Type Conversion16/1
  Bit Shift30/1 -> Data Type Conversion15/1
  Bit Shift31/1 -> Data Type Conversion43/1
  Bit Shift32/1 -> Data Type Conversion14/1
  Bit Shift33/1 -> Data Type Conversion42/1
  Data Type Conversion1/1 -> Bit Concat/18
  Data Type Conversion12/1 -> Bit Concat/3
  Data Type Conversion13/1 -> Bit Concat/2
  Data Type Conversion14/1 -> Bit Concat/11
  Data Type Conversion15/1 -> Bit Concat/9
  Data Type Conversion16/1 -> Bit Concat/8
  Data Type Conversion2/1 -> Bit Concat/1
  Data Type Conversion26/1 -> Bit Concat/7
  Data Type Conversion34/1 -> Bit Concat/6
  Data Type Conversion35/1 -> Bit Concat/5
  Data Type Conversion36/1 -> Bit Concat/4
  Data Type Conversion37/1 -> Bit Concat/17
  Data Type Conversion38/1 -> Bit Concat/16
  Data Type Conversion39/1 -> Bit Concat/15
  Data Type Conversion40/1 -> Bit Concat/14
  Data Type Conversion41/1 -> Bit Concat/13
  Data Type Conversion42/1 -> Bit Concat/12
  Data Type Conversion43/1 -> Bit Concat/10
  Data Type Conversion44/1 -> Out1/1

== system gm_DUALportRAMinterface_v3/PL/to_uint32_6 ==
  u_port : Inport  OutDataTypeStr=fixdt(1, 33, 15)  PortDimensions=1  SampleTime=3.00000003e-08
  Bit Concat : hdlsllib/Logic and Bit Operations/Bit Concat  numInputs=18
  Bit Shift1 : hdlsllib/Logic and Bit Operations/Bit Shift  mode=Shift Left Logical  N=15
  Bit Shift19 : hdlsllib/Logic and Bit Operations/Bit Shift  mode=Shift Left Logical  N=1
  Bit Shift2 : hdlsllib/Logic and Bit Operations/Bit Shift  mode=Shift Right Logical  N=16
  Bit Shift20 : hdlsllib/Logic and Bit Operations/Bit Shift  mode=Shift Left Logical  N=10
  Bit Shift21 : hdlsllib/Logic and Bit Operations/Bit Shift  mode=Shift Right Logical  N=1
  Bit Shift22 : hdlsllib/Logic and Bit Operations/Bit Shift  mode=Shift Left Logical  N=11
  Bit Shift23 : hdlsllib/Logic and Bit Operations/Bit Shift  mode=Shift Left Logical  N=12
  Bit Shift24 : hdlsllib/Logic and Bit Operations/Bit Shift  mode=Shift Left Logical  N=13
  Bit Shift25 : hdlsllib/Logic and Bit Operations/Bit Shift  mode=Shift Left Logical  N=14
  Bit Shift26 : hdlsllib/Logic and Bit Operations/Bit Shift  mode=Shift Left Logical  N=2
  Bit Shift27 : hdlsllib/Logic and Bit Operations/Bit Shift  mode=Shift Left Logical  N=3
  Bit Shift28 : hdlsllib/Logic and Bit Operations/Bit Shift  mode=Shift Left Logical  N=4
  Bit Shift29 : hdlsllib/Logic and Bit Operations/Bit Shift  mode=Shift Left Logical  N=5
  Bit Shift30 : hdlsllib/Logic and Bit Operations/Bit Shift  mode=Shift Left Logical  N=6
  Bit Shift31 : hdlsllib/Logic and Bit Operations/Bit Shift  mode=Shift Left Logical  N=7
  Bit Shift32 : hdlsllib/Logic and Bit Operations/Bit Shift  mode=Shift Left Logical  N=8
  Bit Shift33 : hdlsllib/Logic and Bit Operations/Bit Shift  mode=Shift Left Logical  N=9
  Data Type Conversion{1..2,12..16,26,34..43} (18 alike) : DataTypeConversion  OutDataTypeStr=fixdt(0,1,0)  SaturateOnIntegerOverflow=off  RndMeth=Floor
  Data Type Conversion44 : DataTypeConversion  OutDataTypeStr=uint32  SaturateOnIntegerOverflow=off  RndMeth=Floor
  Out1 : Outport  SampleTime=3.00000003e-08
  wires:
  u_port/1 -> Data Type Conversion12/1, Bit Shift33/1, Bit Shift32/1, Bit Shift31/1, Bit Shift30/1, Bit Shift29/1, Bit Shift28/1, Bit Shift27/1, Bit Shift26/1, Bit Shift25/1, Bit Shift24/1, Bit Shift23/1, Bit Shift22/1, Bit Shift21/1, Bit Shift20/1, Bit Shift2/1, Bit Shift19/1, Bit Shift1/1
  Bit Concat/1 -> Data Type Conversion44/1
  Bit Shift1/1 -> Data Type Conversion1/1
  Bit Shift19/1 -> Data Type Conversion36/1
  Bit Shift2/1 -> Data Type Conversion2/1
  Bit Shift20/1 -> Data Type Conversion41/1
  Bit Shift21/1 -> Data Type Conversion13/1
  Bit Shift22/1 -> Data Type Conversion40/1
  Bit Shift23/1 -> Data Type Conversion39/1
  Bit Shift24/1 -> Data Type Conversion38/1
  Bit Shift25/1 -> Data Type Conversion37/1
  Bit Shift26/1 -> Data Type Conversion35/1
  Bit Shift27/1 -> Data Type Conversion34/1
  Bit Shift28/1 -> Data Type Conversion26/1
  Bit Shift29/1 -> Data Type Conversion16/1
  Bit Shift30/1 -> Data Type Conversion15/1
  Bit Shift31/1 -> Data Type Conversion43/1
  Bit Shift32/1 -> Data Type Conversion14/1
  Bit Shift33/1 -> Data Type Conversion42/1
  Data Type Conversion1/1 -> Bit Concat/18
  Data Type Conversion12/1 -> Bit Concat/3
  Data Type Conversion13/1 -> Bit Concat/2
  Data Type Conversion14/1 -> Bit Concat/11
  Data Type Conversion15/1 -> Bit Concat/9
  Data Type Conversion16/1 -> Bit Concat/8
  Data Type Conversion2/1 -> Bit Concat/1
  Data Type Conversion26/1 -> Bit Concat/7
  Data Type Conversion34/1 -> Bit Concat/6
  Data Type Conversion35/1 -> Bit Concat/5
  Data Type Conversion36/1 -> Bit Concat/4
  Data Type Conversion37/1 -> Bit Concat/17
  Data Type Conversion38/1 -> Bit Concat/16
  Data Type Conversion39/1 -> Bit Concat/15
  Data Type Conversion40/1 -> Bit Concat/14
  Data Type Conversion41/1 -> Bit Concat/13
  Data Type Conversion42/1 -> Bit Concat/12
  Data Type Conversion43/1 -> Bit Concat/10
  Data Type Conversion44/1 -> Out1/1

== system gm_DUALportRAMinterface_v3/PL/integration_block1/D2 ==
  GAerror : Inport  OutDataTypeStr=fixdt(1, 16, 14)  PortDimensions=1  SampleTime=3.00000003e-08
  push_individual : Inport  Port=2  OutDataTypeStr=boolean  PortDimensions=1  SampleTime=3.00000003e-08
  reset_D2 : Inport  Port=3  OutDataTypeStr=boolean  PortDimensions=1  SampleTime=3.00000003e-08
  Individual_input : Inport  Port=4  OutDataTypeStr=fixdt(1, 33, 15)  PortDimensions=[7]  SampleTime=3.00000003e-08
  Product{,1..5} (6 alike) : Product  Inputs=**  OutDataTypeStr=fixdt(1, 64, 32)  SampleTime=3.00000003e-08
  denom_acc11 : Sum  Inputs=+-  OutDataTypeStr=fixdt(1, 64, 32)  AccumDataTypeStr=fixdt(1, 64, 32)  SampleTime=3.00000003e-08
  denom_acc2 : Sum  Inputs=+-  OutDataTypeStr=fixdt(1, 64, 32)  AccumDataTypeStr=fixdt(1, 64, 32)  SampleTime=3.00000003e-08
  denom_acc3 : Sum  Inputs=+-  OutDataTypeStr=fixdt(1, 64, 32)  AccumDataTypeStr=fixdt(1, 64, 32)  SampleTime=3.00000003e-08
  individual1 : Subsystem
  individual1_term0 : Terminator
  output_cast1 : Subsystem  mask(Buffer/Wire){}
      mask help: Buffer
  reset_sw{,1..6} (7 alike) : Switch  Criteria=u2 > Threshold  Threshold=double(0)  OutDataTypeStr=fixdt(1, 64, 32)  SampleTime=3.00000003e-08  SaturateOnIntegerOverflow=off  InputSameDT=off
  s_nume_acc11 : Sum  OutDataTypeStr=fixdt(1, 64, 32)  AccumDataTypeStr=fixdt(1, 65, 32)  SampleTime=3.00000003e-08
  s_nume_acc2 : Sum  OutDataTypeStr=fixdt(1, 64, 32)  AccumDataTypeStr=fixdt(1, 65, 32)  SampleTime=3.00000003e-08
  s_nume_acc3 : Sum  OutDataTypeStr=fixdt(1, 14, 12)  AccumDataTypeStr=fixdt(1, 65, 32)  SampleTime=3.00000003e-08
  s_state_out11 : Delay  DelayLength=double(1)  InitialCondition=0  SampleTime=3.00000003e-08
  s_state_out2 : Delay  DelayLength=double(1)  InitialCondition=0  SampleTime=3.00000003e-08
  s_state_out3 : Delay  DelayLength=double(1)  InitialCondition=0  SampleTime=3.00000003e-08
  t : Demux  Outputs=7
  zero{,1..6} (7 alike) : Constant  Value="fi(0,1,64,32,\"hex\",\"0000000000000000\")"  OutDataTypeStr=fixdt(1, 64, 32)  SampleTime=3.00000003e-08
  response : Outport  SampleTime=3.00000003e-08
  wires:
  push_individual/1 -> individual1/8(enable)
  reset_D2/1 -> reset_sw3/2, reset_sw2/2, reset_sw1/2, reset_sw/2, reset_sw6/2, reset_sw5/2, reset_sw4/2
  Individual_input/1 -> t/1
  Product3/1 -> reset_sw2/3
  Product4/1 -> reset_sw1/3
  Product5/1 -> reset_sw/3
  denom_acc3/1 -> reset_sw3/3, s_state_out11/1
  individual1/2(a2) -> Product5/2
  individual1/3(a3) -> Product4/2
  individual1/4(a4) -> Product3/2
  output_cast1/1(out) -> response/1
  reset_sw/1 -> s_nume_acc11/2
  reset_sw1/1 -> s_nume_acc2/2
  reset_sw2/1 -> s_nume_acc3/2
  reset_sw3/1 -> s_nume_acc11/1
  s_nume_acc11/1 -> s_nume_acc2/1
  s_nume_acc2/1 -> s_nume_acc3/1
  s_nume_acc3/1 -> output_cast1/1(in)
  s_state_out11/1 -> Product5/1, s_state_out2/1, Product2/1
  s_state_out2/1 -> Product4/1, s_state_out3/1, Product1/1
  s_state_out3/1 -> Product3/1, Product/1
  zero/1 -> reset_sw/1
  zero1/1 -> reset_sw1/1
  zero2/1 -> reset_sw2/1
  zero3/1 -> reset_sw3/1
  individual1/1(score) -> individual1_term0/1
  t/1 -> individual1/1(reg_in)
  t/2 -> individual1/2(reg_in1)
  t/3 -> individual1/3(reg_in2)
  t/4 -> individual1/4(reg_in3)
  t/5 -> individual1/5(reg_in4)
  t/6 -> individual1/6(reg_in5)
  t/7 -> individual1/7(reg_in6)
  individual1/7(b4) -> Product/2
  zero6/1 -> reset_sw4/1
  individual1/6(b3) -> Product1/2
  zero5/1 -> reset_sw5/1
  individual1/5(b2) -> Product2/2
  zero4/1 -> reset_sw6/1
  GAerror/1 -> denom_acc11/1
  Product/1 -> reset_sw4/3
  reset_sw4/1 -> denom_acc3/2
  Product1/1 -> reset_sw5/3
  reset_sw5/1 -> denom_acc2/2
  Product2/1 -> reset_sw6/3
  reset_sw6/1 -> denom_acc11/2
  denom_acc11/1 -> denom_acc2/1
  denom_acc2/1 -> denom_acc3/1
